simulink model "Control_test"  (R2023a)
settings: Solver=VariableStepAuto  StartTime=0.0  StopTime=100  RelTol=1e-3
libraries: SignalEditorBlockLib x1
settings Model: Creator=tatyn  LastModifiedBy=tatyn

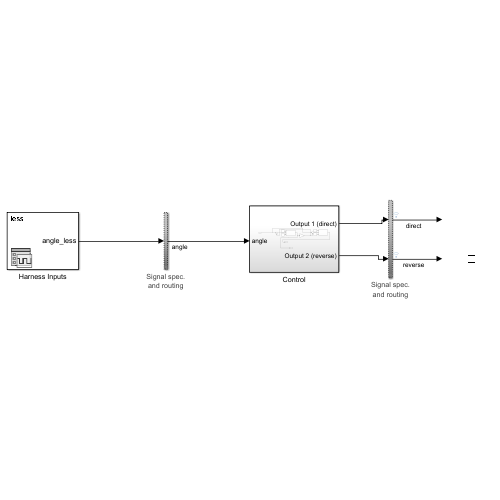
[thumbnail: Simulink's stored preview of the top-level diagram]
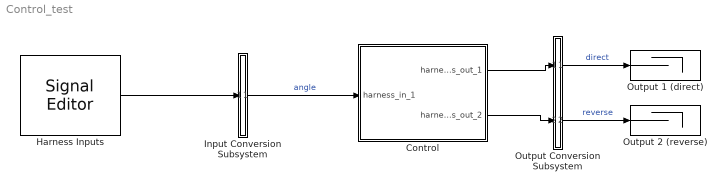
== system Control_test ==
  Control : Subsystem  Tag=__SL_testing_harness_stub_
  Harness Inputs : SignalEditorBlockLib/Signal Editor  FileName=C:\Users\tatyn\Desktop\lab6\privod\Tests\Control_test_HarnessInputs.mat  ActiveScenario=less  ActiveSignal=angle_less  IsBus=off  OutputBusObjectStr=Bus: BusObject  SampleTime=0  Interpolate=off  ZeroCross=off  OutputAfterFinalValue=Setting to zero  Unit=inherit  PreserveSignalName=on  ApplySigPropsToAllScenarios=on
  Input Conversion Subsystem : Subsystem  Tag=__SLT_ICS__  Description=|
      | Signal spec.
      | and routing
      settings: AttributesFormatString=%<Description>
  Output Conversion Subsystem : Subsystem  Tag=__SLT_OCS__  Description=|
      | Signal spec.
      | and routing
      settings: AttributesFormatString=%<Description>
  Output 1 (direct) : Terminator
  Output 2 (reverse) : Terminator
  wires:
  Harness Inputs/1 -> Input Conversion Subsystem/1(Inport_1)
  Output Conversion Subsystem/1(Outport_1) -> Output 1 (direct)/1  "direct"
  Output Conversion Subsystem/2(Outport_2) -> Output 2 (reverse)/1  "reverse"
  Input Conversion Subsystem/1(Outport_1) -> Control/1(harness_in_1)  "angle"
  Control/1(harness_out_1) -> Output Conversion Subsystem/1(Inport_1)
  Control/2(harness_out_2) -> Output Conversion Subsystem/2(Inport_2)

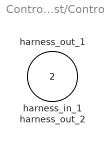
== system Control_test/Control ==
  harness_in_1 : Inport
  harness_out_1 : Outport
  harness_out_2 : Outport  Port=2

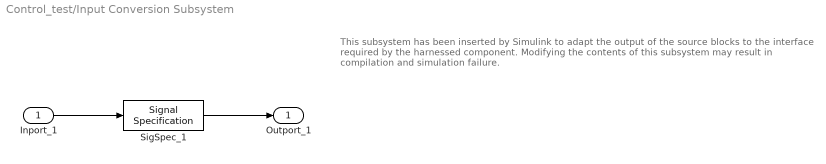
== system Control_test/Input Conversion Subsystem ==
  note: This subsystem has been inserted by Simulink to adapt the output of the source blocks to the interface required by the harnessed component.
      |  Modifying the contents of this subsystem may result in compilation and simulation failure.
  Inport_1 : Inport
  SigSpec_1 : SignalSpecification  OutDataTypeStr=double  Unit=rad  Dimensions=[1]  SampleTime=[0, 0]
  Outport_1 : Outport
  wires:
  SigSpec_1/1 -> Outport_1/1
  Inport_1/1 -> SigSpec_1/1

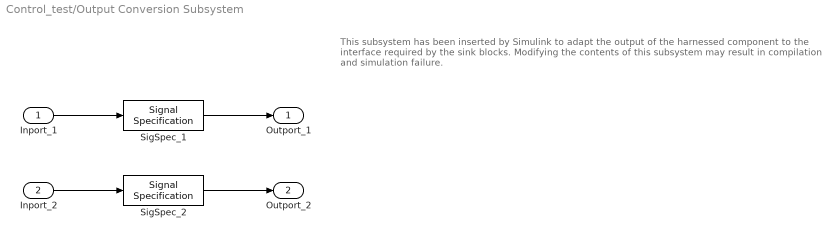
== system Control_test/Output Conversion Subsystem ==
  note: This subsystem has been inserted by Simulink to adapt the output of the harnessed component to the interface required by the sink blocks.
      |  Modifying the contents of this subsystem may result in compilation and simulation failure.
  Inport_1 : Inport
  Inport_2 : Inport  Port=2
  SigSpec_1 : SignalSpecification  OutDataTypeStr=double  Unit=1  Dimensions=[1]
  SigSpec_2 : SignalSpecification  OutDataTypeStr=double  Unit=1  Dimensions=[1]
  Outport_1 : Outport
  Outport_2 : Outport  Port=2
  wires:
  Inport_1/1 -> SigSpec_1/1
  SigSpec_1/1 -> Outport_1/1
  Inport_2/1 -> SigSpec_2/1
  SigSpec_2/1 -> Outport_2/1
